simulink model "ekf_1d"  (R2024b)
settings: Solver=VariableStepAuto  StartTime=0.0  StopTime=10.0  RelTol=1e-3
undefined symbols (not defined in the file): DiscIntNeverNeededParam
settings Model: Creator=rasim  LastModifiedBy=rasim

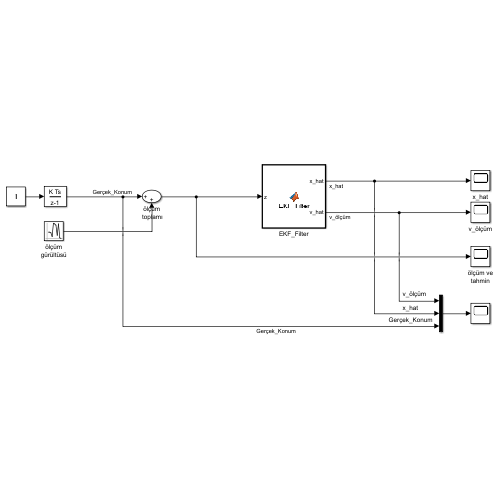
[thumbnail: Simulink's stored preview of the top-level diagram]
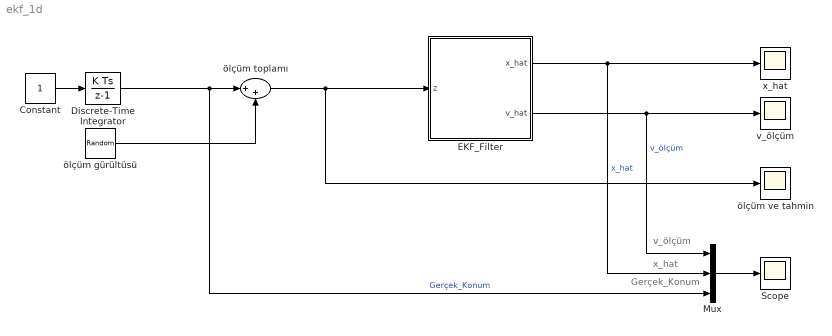
== system ekf_1d ==
  note: Gerçek_Konum
  note: x_hat
  note: v_ölçüm
  Constant : Constant
  Discrete-Time Integrator : DiscreteIntegrator  ICPrevOutput=DiscIntNeverNeededParam  ICPrevScaledInput=DiscIntNeverNeededParam
  EKF_Filter : MATLAB Function  TreatAsAtomicUnit=on
  Mux : Mux  Inputs=3
  Scope : Scope
  v_ölçüm : Scope
  x_hat : Scope
  ölçüm toplamı : Sum  Inputs=|++
  ölçüm gürültüsü : RandomNumber  Variance=30  SampleTime=0.1
  ölçüm ve tahmin : Scope
  wires:
  Constant/1 -> Discrete-Time Integrator/1
  Discrete-Time Integrator/1 -> Mux/3, ölçüm toplamı/1  "Gerçek_Konum"
  ölçüm gürültüsü/1 -> ölçüm toplamı/2
  ölçüm toplamı/1 -> ölçüm ve tahmin/1, EKF_Filter/1(z)
  EKF_Filter/1(x_hat) -> x_hat/1, Mux/2  "x_hat"
  EKF_Filter/2(v_hat) -> v_ölçüm/1, Mux/1  "v_ölçüm"
  Mux/1 -> Scope/1

== matlab function ekf_1d/EKF_Filter ==
  data: z input; x_hat output; v_hat output
function [x_hat, v_hat] = EKF_Filter(z)

% Kalıcı değişkenler
persistent x P A H Q R

if isempty(x)
    dt = 1;
    x = [0; 1];           % Başlangıç: konum=0, hız=1
    P = eye(2);           % Başlangıç kovaryans
    A = [1 dt; 0 1];      % Durum geçiş matrisi
    H = [1 0];            % Ölçüm matrisi
    Q = 0.01 * eye(2);    % Süreç gürültüsü
    R = 1;                % Ölçüm gürültüsü
end

% Tahmin
x_pred = A * x;
P_pred = A * P * A' + Q;

% Güncelleme
y = z - H * x_pred;             % Artık
S = H * P_pred * H' + R;        % Artık kovaryansı
K = P_pred * H' / S;            % Kalman kazancı

x = x_pred + K * y;             % Durum tahmini
P = (eye(2) - K * H) * P_pred;  % Kovaryans güncellemesi

x_hat = x(1);   % Tahmin edilen konum
v_hat = x(2);   % Tahmin edilen hız
